simulink model "Errore_lab1_PositionPIDController"  (R2020b)
settings: Solver=VariableStepAuto  StartTime=0.0  StopTime=10.0  RelTol=1e-3
undefined symbols (not defined in the file): K_D, K_I, K_P, sens, stepAmplitude, T_L
settings Model: Creator=Musta  LastModifiedBy=Musta

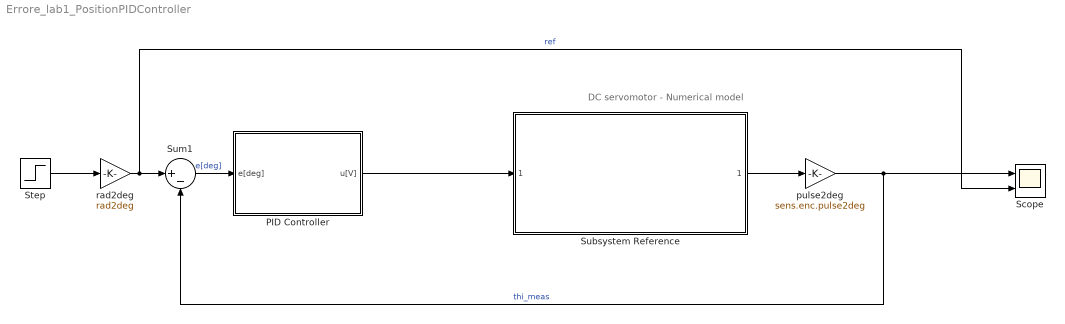
== system Errore_lab1_PositionPIDController ==
  note: DC servomotor - Numerical model
  PID Controller : Subsystem
  Scope : Scope  NumInputPorts=2
  Step : Step  Time=0  After=stepAmplitude  SampleTime=0
  Subsystem Reference : Subsystem  ReferencedSubsystem=plant_Model
  Sum1 : Sum  Inputs=|+-
  pulse2deg : Gain  Gain=sens.enc.pulse2deg
  rad2deg : Gain  Gain=rad2deg
  wires:
  rad2deg/1 -> Scope/2, Sum1/1  "ref"
  Subsystem Reference/1 -> pulse2deg/1
  PID Controller/1(u[V]) -> Subsystem Reference/1
  Sum1/1 -> PID Controller/1(e[deg])  "e[deg]"
  Step/1 -> rad2deg/1
  pulse2deg/1 -> Sum1/2, Scope/1  "thi_meas"

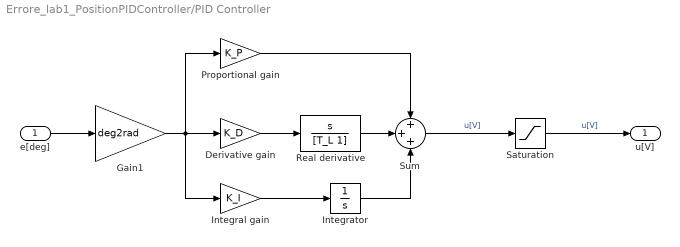
== system Errore_lab1_PositionPIDController/PID Controller ==
  e[deg] : Inport
  Derivative gain : Gain  Gain=K_D
  Gain1 : Gain  Gain=deg2rad
  Integral gain : Gain  Gain=K_I
  Integrator : Integrator
  Proportional gain : Gain  Gain=K_P
  Real derivative : TransferFcn  Numerator=[1 0]  Denominator=[T_L 1]
  Saturation : Saturate  UpperLimit=10  LowerLimit=-10
  Sum : Sum  Inputs=+++
  u[V] : Outport
  wires:
  e[deg]/1 -> Gain1/1
  Real derivative/1 -> Sum/2
  Gain1/1 -> Derivative gain/1, Integral gain/1, Proportional gain/1
  Proportional gain/1 -> Sum/1
  Integrator/1 -> Sum/3
  Derivative gain/1 -> Real derivative/1
  Sum/1 -> Saturation/1  "u[V]"
  Saturation/1 -> u[V]/1  "u[V]"
  Integral gain/1 -> Integrator/1
